simulink subsystem "Battery_Module"  (R2021b)
settings: Solver=VariableStepAuto  StartTime=0.0  StopTime=10.0  RelTol=1e-3
libraries: nesl_utility x6
settings Model: Creator=tshintai  LastModifiedBy=tshintai

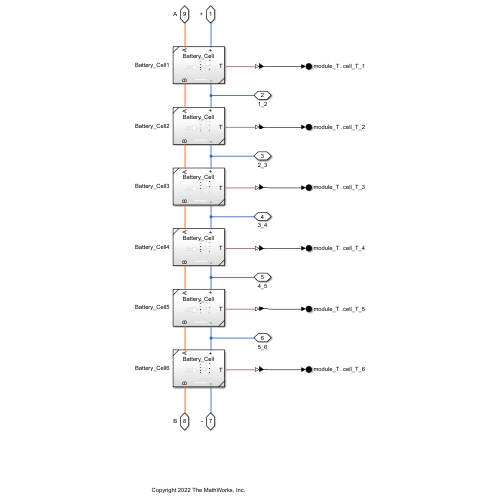
[thumbnail: Simulink's stored preview of the top-level diagram]
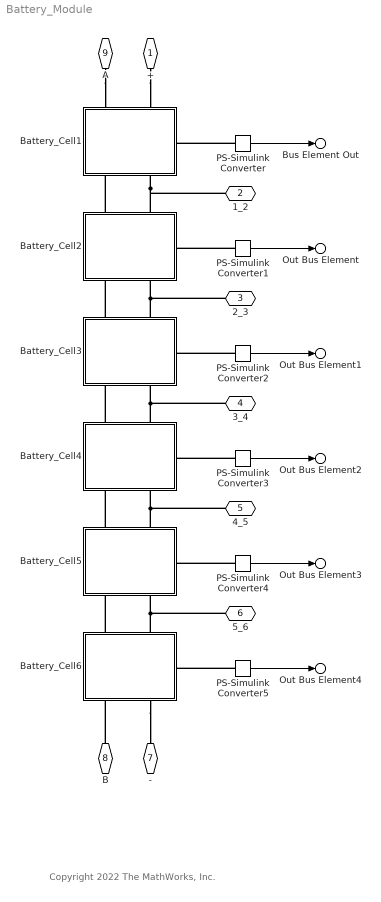
== system Battery_Module ==
  note: Copyright 2022 The MathWorks, Inc.
  Battery_Cell{1..6} (6 alike) : Subsystem  ReferencedSubsystem=Battery_Cell
      settings: PortSchema="{\"entries\":[{\"content\":{\"sides\":[{\"content\":{\"connectorIds\":[]},\"type\":\"ConnectorPlacement.EquallySpacedRectSide\",\"uuid\":\"33b27dc5-87b7-4bec-a7ec-b54dd59365bf\"},{\"content\":{\"connectorIds\":[\"RConn1\"],\"side\":\"RIGHT\"},\"type\":\"ConnectorPlacement.EquallySpacedRectSide\",\"uuid\":\"0950a7a6-977c-48dc-b545-1b58ae61d99f\"},{\"content\":{\"connectorIds\":[\"LConn1\",\"LConn2\"],\"side\":\"TOP\"},\"type\":\"ConnectorPlacement.EquallySpacedRectSide\",\"uuid\":\"c35d4de5-9023-4aa1-a1b5-51c284742a56\"},{\"content\":{\"connectorIds\":[\"RConn2\",\"RConn3\"],\"side\":\"BOTTOM\"},\"type\":\"ConnectorPlacement.EquallySpacedRectSide\",\"uuid\":\"06cf3f50-4349-498f-9f72-c49451d97ba0\"}]},\"type\":\"ConnectorPlacement.EquallySpacedConnector\",\"uuid\":\"dda559ed-5d24-4b24-a833-e9b2314532a8\"}],\"packageUris\":[\"http://schema.mathworks.com/mf0/Connector/R2020b\"],\"version\":\"1.0\"}"
  PS-Simulink Converter{,1..5} (6 alike) : nesl_utility/PS-Simulink Converter  PhysicalDomain=network_engine_domain  SubClassName=ps_output  LeftPortType=input  RightPortType=output  PseudoPeriodic=off  Frequencies=[]  Unit=inherit  AffineConversion=off
      settings: SourceProductBaseCode=PW,SS
  + : PMIOPort  Side=Right
  1_2 : PMIOPort  Port=2  Side=Right
  2_3 : PMIOPort  Port=3  Side=Right
  3_4 : PMIOPort  Port=4  Side=Right
  4_5 : PMIOPort  Port=5  Side=Right
  5_6 : PMIOPort  Port=6  Side=Right
  - : PMIOPort  Port=7  Side=Right
  B : PMIOPort  Port=8  Side=Right
  A : PMIOPort  Port=9  Side=Right
  Bus Element Out : Outport  PortName=module_T  Element=cell_T_1
  Out Bus Element : Outport  PortName=module_T  Element=cell_T_2
  Out Bus Element1 : Outport  PortName=module_T  Element=cell_T_3
  Out Bus Element2 : Outport  PortName=module_T  Element=cell_T_4
  Out Bus Element3 : Outport  PortName=module_T  Element=cell_T_5
  Out Bus Element4 : Outport  PortName=module_T  Element=cell_T_6
  wires:
  PS-Simulink Converter4/1 -> Out Bus Element3/1
  PS-Simulink Converter1/1 -> Out Bus Element/1
  PS-Simulink Converter/1 -> Bus Element Out/1
  PS-Simulink Converter5/1 -> Out Bus Element4/1
  PS-Simulink Converter2/1 -> Out Bus Element1/1
  PS-Simulink Converter3/1 -> Out Bus Element2/1
  connections:
  2_3/RConn1 -- Battery_Cell3/LConn2 -- Battery_Cell2/RConn3
  3_4/RConn1 -- Battery_Cell4/LConn2 -- Battery_Cell3/RConn3
  5_6/RConn1 -- Battery_Cell6/LConn2 -- Battery_Cell5/RConn3
  Battery_Cell5/LConn2 -- Battery_Cell4/RConn3 -- 4_5/RConn1
  Battery_Cell1/RConn3 -- Battery_Cell2/LConn2 -- 1_2/RConn1
  PS-Simulink Converter/LConn1 -- Battery_Cell1/RConn1
  Battery_Cell5/LConn1 -- Battery_Cell4/RConn2
  PS-Simulink Converter4/LConn1 -- Battery_Cell5/RConn1
  PS-Simulink Converter1/LConn1 -- Battery_Cell2/RConn1
  B/RConn1 -- Battery_Cell6/RConn2
  Battery_Cell2/LConn1 -- Battery_Cell1/RConn2
  PS-Simulink Converter5/LConn1 -- Battery_Cell6/RConn1
  Battery_Cell6/LConn1 -- Battery_Cell5/RConn2
  PS-Simulink Converter3/LConn1 -- Battery_Cell4/RConn1
  PS-Simulink Converter2/LConn1 -- Battery_Cell3/RConn1
  Battery_Cell4/LConn1 -- Battery_Cell3/RConn2
  +/RConn1 -- Battery_Cell1/LConn2
  Battery_Cell3/LConn1 -- Battery_Cell2/RConn2
  A/RConn1 -- Battery_Cell1/LConn1
  Battery_Cell6/RConn3 -- -/RConn1
